simulink model "pd_control"  (R2024b)
settings: Solver=VariableStepAuto  StartTime=0.0  StopTime=10.0  RelTol=1e-3
settings Model: Creator=bsb  LastModifiedBy=bsb
settings SolverCC: AlgebraicLoopSolver=TrustRegion
settings DebuggingCC: UnconnectedInputMsg=warning  UnconnectedOutputMsg=warning  UnconnectedLineMsg=warning
settings ModelReferenceCC: EnableRefExpFcnMdlSchedulingChecks=on
settings RTWCC: GPUComputeCapability=3.5

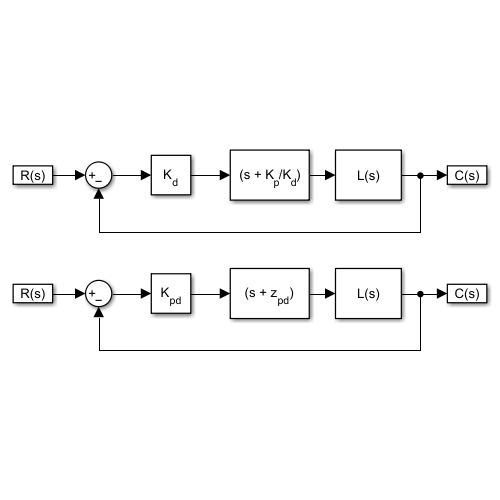
[thumbnail: Simulink's stored preview of the top-level diagram]
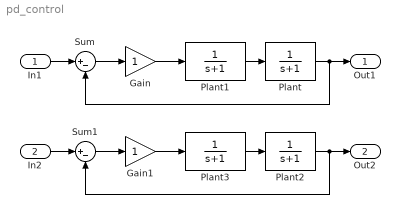
== system pd_control ==
  In1 : Inport
      mask Display: disp('R(s)')
  In2 : Inport  Port=2
      mask Display: disp('R(s)')
  Gain : Gain
      mask Display: disp('K_d','interpreter','tex')
  Gain1 : Gain
      mask Display: disp('K_{pd}','interpreter','tex')
  Plant{,1..3} (4 alike) : TransferFcn  Numerator=1  Denominator=[1 1]  ContinuousStateAttributes='theta'
      Plant mask Display: disp('L(s)')
      Plant1 mask Display: disp('(s + K_p/K_d)','interpreter','tex')
      Plant2 mask Display: disp('L(s)')
      Plant3 mask Display: disp('(s + z_{pd})','interpreter','tex')
  Sum : Sum  Inputs=|+-
  Sum1 : Sum  Inputs=|+-
  Out1 : Outport
      mask Display: disp('C(s)')
  Out2 : Outport  Port=2
      mask Display: disp('C(s)')
  wires:
  Plant/1 -> Sum/2, Out1/1
  Gain/1 -> Plant1/1
  In1/1 -> Sum/1
  Sum/1 -> Gain/1
  Plant1/1 -> Plant/1
  Sum1/1 -> Gain1/1
  In2/1 -> Sum1/1
  Plant3/1 -> Plant2/1
  Gain1/1 -> Plant3/1
  Plant2/1 -> Sum1/2, Out2/1
